simulink model "Hybrid"  (R2024b)
settings: Solver=VariableStepAuto  StartTime=0.0  StopTime=4000  RelTol=1e-3
undefined symbols (not defined in the file): Acid, Ion, Lead, Lithium
libraries: spsBatteryLib x6, spsCurrentMeasurementLib x2, spsMosfetLib x2, spsSeriesRLCBranchLib x2, spsVoltageMeasurementLib x2, sps_lib x1, spspowerguiLib x1
settings Model: Creator=shiva  LastModifiedBy=shiva

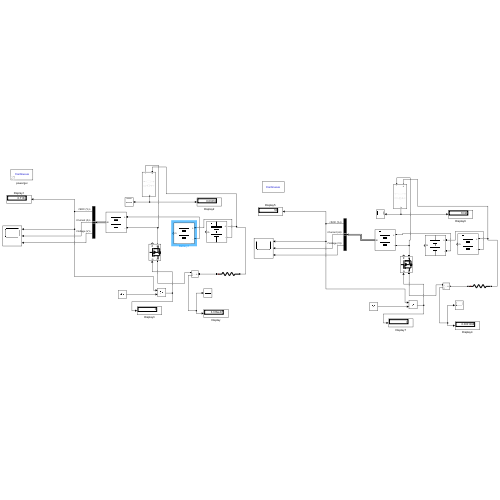
[thumbnail: Simulink's stored preview of the top-level diagram]
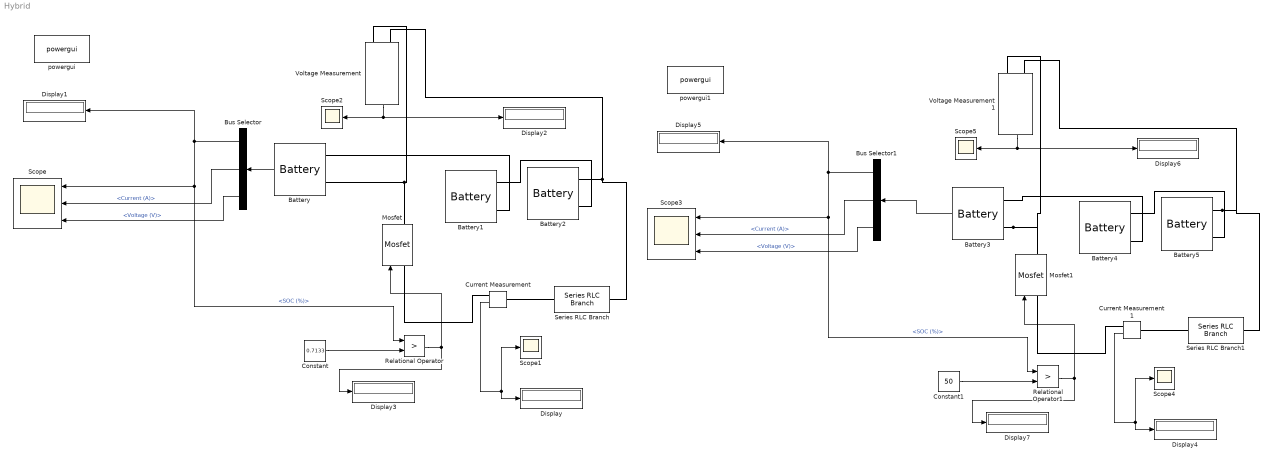
== system Hybrid ==
  Battery : spsBatteryLib/Battery  BatType=Lithium-Ion  NomV=3.7  NomQ=2.6  SOC=96  Batt_Tr=30  PresetModel=on  MaxQ=2.6  MinV=2.775  FullV=4.3068  Dis_rate=1.1304  R=0.014231  Normal_OP=2.3513  expZone="[3.9974     0.12774]"
  Battery1 : spsBatteryLib/Battery  BatType=Lithium-Ion  NomV=3.7  NomQ=2.6  SOC=96  Batt_Tr=30  PresetModel=on  MaxQ=2.6  MinV=2.775  FullV=4.3068  Dis_rate=1.1304  R=0.014231  Normal_OP=2.3513  expZone="[3.9974     0.12774]"
  Battery2 : spsBatteryLib/Battery  BatType=Lithium-Ion  NomV=3.7  NomQ=2.6  SOC=96  Batt_Tr=30  PresetModel=on  MaxQ=2.6  MinV=2.775  FullV=4.3068  Dis_rate=1.1304  R=0.014231  Normal_OP=2.3513  expZone="[3.9974     0.12774]"
  Battery3 : spsBatteryLib/Battery  BatType=Lead-Acid  NomV=3.7  NomQ=2.6  SOC=94  Batt_Tr=30  PresetModel=on  MaxQ=2.7083  MinV=2.775  FullV=4.0286  Dis_rate=0.52  R=0.014231  Normal_OP=0.80672  expZone="[3.7669   0.0086667]"
  Battery4 : spsBatteryLib/Battery  BatType=Lead-Acid  NomV=3.7  NomQ=2.6  SOC=94  Batt_Tr=30  PresetModel=on  MaxQ=2.7083  MinV=2.775  FullV=4.0286  Dis_rate=0.52  R=0.014231  Normal_OP=0.80672  expZone="[3.7669   0.0086667]"
  Battery5 : spsBatteryLib/Battery  BatType=Lead-Acid  NomV=3.7  NomQ=2.6  SOC=96  Batt_Tr=30  PresetModel=on  MaxQ=2.7083  MinV=2.775  FullV=4.0286  Dis_rate=0.52  R=0.014231  Normal_OP=0.80672  expZone="[3.7669   0.0086667]"
  Bus Selector : BusSelector  OutputSignals=SOC (%),Current (A),Voltage (V)
  Bus Selector1 : BusSelector  OutputSignals=SOC (%),Current (A),Voltage (V)
  Constant : Constant  Value=0.7133
  Constant1 : Constant  Value=50
  Current Measurement : spsCurrentMeasurementLib/Current Measurement  PhasorSimulation=off  OutputType=Complex  PSBequivalent=0
  Current Measurement1 : spsCurrentMeasurementLib/Current Measurement  PhasorSimulation=off  OutputType=Complex  PSBequivalent=0
  Display{,1..7} (8 alike) : Display
  Mosfet : spsMosfetLib/Mosfet  Ron=0.1  Lon=0  Rd=0.01  Vfd=0  IC=0  Rs=1e5  Cs=inf  Measurements=on
  Mosfet1 : spsMosfetLib/Mosfet  Ron=0.1  Lon=0  Rd=0.01  Vfd=0  IC=0  Rs=1e5  Cs=inf  Measurements=on
  Relational Operator : RelationalOperator  Operator=>  OutDataTypeStr=boolean  RndMeth=Simplest  InputSameDT=off
  Relational Operator1 : RelationalOperator  Operator=>  OutDataTypeStr=boolean  RndMeth=Simplest  InputSameDT=off
  Scope : Scope  NumInputPorts=3
  Scope{1..2,4..5} (4 alike) : Scope
  Scope3 : Scope  NumInputPorts=3
  Series RLC Branch : spsSeriesRLCBranchLib/Series RLC Branch  LConnTagsString=__new0  RConnTagsString=__new0  BranchType=R  Resistance=4.4  Inductance=1e-3  SetiL0=off  InitialCurrent=0  Capacitance=1e-6  Setx0=off  InitialVoltage=0  Measurements=None
  Series RLC Branch1 : spsSeriesRLCBranchLib/Series RLC Branch  LConnTagsString=__new0  RConnTagsString=__new0  BranchType=R  Resistance=4.4  Inductance=1e-3  SetiL0=off  InitialCurrent=0  Capacitance=1e-6  Setx0=off  InitialVoltage=0  Measurements=None
  Voltage Measurement : spsVoltageMeasurementLib/Voltage Measurement  PhasorSimulation=off  OutputType=Complex  PSBequivalent=0
  Voltage Measurement1 : spsVoltageMeasurementLib/Voltage Measurement  PhasorSimulation=off  OutputType=Complex  PSBequivalent=0
  powergui : sps_lib/powergui  Priority=1  SimulationMode=Continuous  SampleTime=50e-6  frequency=60  Iterations=50  frequencyindice=0  Pbase=100e6  ErrMax=1e-4  UnitsV=kV  UnitsW=MW  buscounter=0  FunctionMessages=off  echomessages=off  EnableUseOfTLC=off  CurrentSourceSwitches=off  DisableSnubberDevices=off  DisableRonSwitches=off  DisableVfSwitches=off  DisplayEquations=off  AutomaticDiscreteSolvers=off  SolverType=Tustin/Backward Euler (TBE)  Interpol=off  ExternalGateDelay=off  methode=off  Ts=100  x0status=blocks  SPID=on  SwTol=0  HookPort=off  NonlinearTolerance=1e-4  nMaxIteration=100  ContinueOnMaxIteration=off  RestoreLinks=warning  ResistiveCurrentMeasurement=off  Frange=[0:2:500]  Ylog=off  Xlog=on  ShowGrid=off  save=off  variable=ZData  structure=0  ZoomFFT=off  StartTime=0.0  cycles=1  DisplayStyle=1  fundamental=60  FreqAxis=off  MaxFrequency=1000  frequencyindicesteady=1  RmsSteady=1  display=off
  powergui1 : spspowerguiLib/powergui  Priority=1  SimulationMode=Continuous  SampleTime=50e-6  frequency=60  Iterations=50  frequencyindice=0  Pbase=100e6  ErrMax=1e-4  UnitsV=kV  UnitsW=MW  buscounter=0  FunctionMessages=off  echomessages=off  EnableUseOfTLC=off  CurrentSourceSwitches=off  DisableSnubberDevices=off  DisableRonSwitches=off  DisableVfSwitches=off  DisplayEquations=off  AutomaticDiscreteSolvers=off  SolverType=Tustin/Backward Euler (TBE)  Interpol=off  ExternalGateDelay=off  methode=off  Ts=100  x0status=blocks  SPID=on  SwTol=0  HookPort=off  NonlinearTolerance=1e-4  nMaxIteration=100  ContinueOnMaxIteration=off  RestoreLinks=warning  ResistiveCurrentMeasurement=off  Frange=[0:2:500]  Ylog=off  Xlog=on  ShowGrid=off  save=off  variable=ZData  structure=0  ZoomFFT=off  StartTime=0.0  cycles=1  DisplayStyle=1  fundamental=60  FreqAxis=off  MaxFrequency=1000  frequencyindicesteady=1  RmsSteady=1  display=off
  wires:
  Relational Operator/1 -> Mosfet/1, Display3/1
  Constant/1 -> Relational Operator/2
  Bus Selector/1 -> Relational Operator/1, Scope/1, Display1/1  "<SOC (%)>"
  Bus Selector/2 -> Scope/2  "<Current (A)>"
  Bus Selector/3 -> Scope/3  "<Voltage (V)>"
  Current Measurement/1 -> Display/1, Scope1/1
  Voltage Measurement/1 -> Display2/1, Scope2/1
  Battery/1 -> Bus Selector/1
  Battery3/1 -> Bus Selector1/1
  Current Measurement1/1 -> Display4/1, Scope4/1
  Bus Selector1/1 -> Relational Operator1/1, Scope3/1, Display5/1  "<SOC (%)>"
  Relational Operator1/1 -> Mosfet1/1, Display7/1
  Bus Selector1/3 -> Scope3/3  "<Voltage (V)>"
  Constant1/1 -> Relational Operator1/2
  Voltage Measurement1/1 -> Display6/1, Scope5/1
  Bus Selector1/2 -> Scope3/2  "<Current (A)>"
  connections:
  Current Measurement/LConn1 -- Series RLC Branch/LConn1
  Mosfet/LConn1 -- Current Measurement/RConn1
  Battery1/LConn2 -- Battery/LConn1
  Battery1/LConn1 -- Battery2/LConn2
  Mosfet/RConn1 -- Voltage Measurement/LConn2 -- Battery/LConn2
  Series RLC Branch/RConn1 -- Voltage Measurement/LConn1 -- Battery2/LConn1
  Battery3/LConn2 -- Voltage Measurement1/LConn2 -- Mosfet1/RConn1
  Battery5/LConn1 -- Series RLC Branch1/RConn1 -- Voltage Measurement1/LConn1
  Battery4/LConn1 -- Battery5/LConn2
  Current Measurement1/LConn1 -- Series RLC Branch1/LConn1
  Battery4/LConn2 -- Battery3/LConn1
  Mosfet1/LConn1 -- Current Measurement1/RConn1
